simulink model "verification_template"  (R2014b)
settings: Solver=ode45  StartTime=0.0  StopTime=10.0  RelTol=1e-3
settings Model: Creator=Romain  LastModifiedBy=Romain
settings DebuggingCC: UnderspecifiedInitializationDetection=Classic  MergeDetectMultiDrivingBlocksExec=none  SolverPrmCheckMsg=none

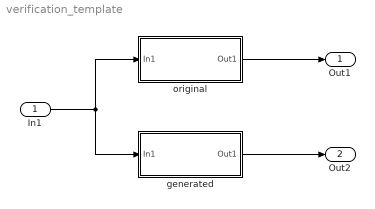
== system verification_template ==
  In1 : Inport  OutDataTypeStr=double
  generated : Subsystem
  original : Subsystem
  Out1 : Outport
  Out2 : Outport  Port=2
  wires:
  In1/1 -> generated/1(In1), original/1(In1)
  original/1(Out1) -> Out1/1
  generated/1(Out1) -> Out2/1

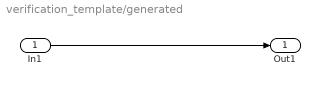
== system verification_template/generated ==
  In1 : Inport
  Out1 : Outport
  wires:
  In1/1 -> Out1/1

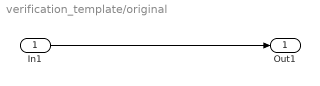
== system verification_template/original ==
  In1 : Inport
  Out1 : Outport
  wires:
  In1/1 -> Out1/1
